simulink model "SAD_testControl"  (R2023b)
settings: Solver=ode8  StartTime=0  StopTime=tf  FixedStep=t_step  RelTol=1e-3
values from neighbouring files (symbols this model uses):
  A_1 = area_face(1)    [SAD_project_code.m]
  A_2 = area_face(2)    [SAD_project_code.m]
  A_3 = area_face(3)    [SAD_project_code.m]
  A_4 = area_face(4)    [SAD_project_code.m]
  A_5 = area_face(5)    [SAD_project_code.m]
  A_6 = area_face(6)    [SAD_project_code.m]
  DCM_eci_per = rotationMatrix(rad2deg(i),rad2deg(OM), rad2deg(om))    [SAD_project_code.m]
  e = 0.0011241    [SAD_project_code.m]
  FS = 50000e-9    (= 5e-05)    [SAD_project_code.m]
  H0 = [g_10 g_11 h_11]'    [SAD_project_code.m]
  h_r_0 = [0,0,0]'    [SAD_project_code.m]
  horizon_cone_limit = deg2rad(70)    [SAD_project_code.m]
  I = 5/12.*diag([Ix Iy Iz])    [SAD_project_code.m]
  i = deg2rad(97.55)    [SAD_project_code.m]
  I_inv = inv(I)    [SAD_project_code.m]
  I_vector_RW = [I_RW I_RW I_RW]'    [SAD_project_code.m]
  inc_tot = sqrt(inc_lin^2 + inc_acc^2)    [SAD_project_code.m]
  InitialTrueAnomalyOfEarth = 0    [SAD_project_code.m]
  j_b = [0.001 0.005 0.001]'    [SAD_project_code.m]
  matrix_RW_config = eye(3)    [SAD_project_code.m]
  matrix_RW_config_inv = inv(matrix_RW_config)    [SAD_project_code.m]
  mu_E = astroConstants(13)    [SAD_project_code.m]
  N_1 = BODY(1,:)    [SAD_project_code.m]
  N_2 = BODY(2,:)    [SAD_project_code.m]
  N_3 = BODY(3,:)    [SAD_project_code.m]
  N_4 = BODY(4,:)    [SAD_project_code.m]
  N_5 = BODY(5,:)    [SAD_project_code.m]
  N_6 = BODY(6,:)    [SAD_project_code.m]
  n_e = sqrt(mu_E/a^3)    [SAD_project_code.m]
  om = deg2rad(206.3209)    [SAD_project_code.m]
  OM = deg2rad(50.7464)    [SAD_project_code.m]
  p = a*(1-e^2)    [SAD_project_code.m]
  q0 = [0.1, -0.7, 0.51, 0.41]    [SAD_project_code.m]
  r_1 = r(1,:)    [SAD_project_code.m]
  r_2 = r(2,:)    [SAD_project_code.m]
  r_3 = r(3,:)    [SAD_project_code.m]
  r_4 = r(4,:)    [SAD_project_code.m]
  r_5 = r(5,:)    [SAD_project_code.m]
  r_6 = r(6,:)    [SAD_project_code.m]
  R_E = astroConstants(23)    [SAD_project_code.m]
  rho_d1 = 0.1    [SAD_project_code.m]
  rho_d2 = 0.1    [SAD_project_code.m]
  rho_d3 = 0.1    [SAD_project_code.m]
  rho_d4 = 0.1    [SAD_project_code.m]
  rho_d5 = 0.1    [SAD_project_code.m]
  rho_d6 = 0.1    [SAD_project_code.m]
  rho_s1 = rho_s(1)    [SAD_project_code.m]
  rho_s2 = rho_s(2)    [SAD_project_code.m]
  rho_s3 = rho_s(3)    [SAD_project_code.m]
  rho_s4 = rho_s(4)    [SAD_project_code.m]
  rho_s5 = rho_s(5)    [SAD_project_code.m]
  rho_s6 = rho_s(6)    [SAD_project_code.m]
  th0 = deg2rad(0)    [SAD_project_code.m]
  ts_sensor = t_step*10    (= 0.1)    [SAD_project_code.m]
  w0 = [wx0 wy0 wz0]'    [SAD_project_code.m]
  w0_RW = [0 0 0]    [SAD_project_code.m]
  w_E = deg2rad(15.04)/60/60    [SAD_project_code.m]
  wMax_RW = 2*pi * RPM_max_RW / 60    (= 527.263967027)    [SAD_project_code.m]
libraries: matrix_library x24, simulink_extras x4, slpidlib x3, sharedtransform x2, simulink x2, vrlib x2, dspinverses x1
(part 1 of 3)
settings Model: Creator=samue  LastModifiedBy=samue

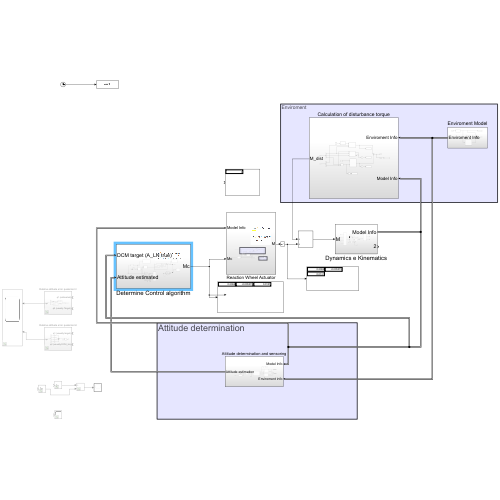
[thumbnail: Simulink's stored preview of the top-level diagram]
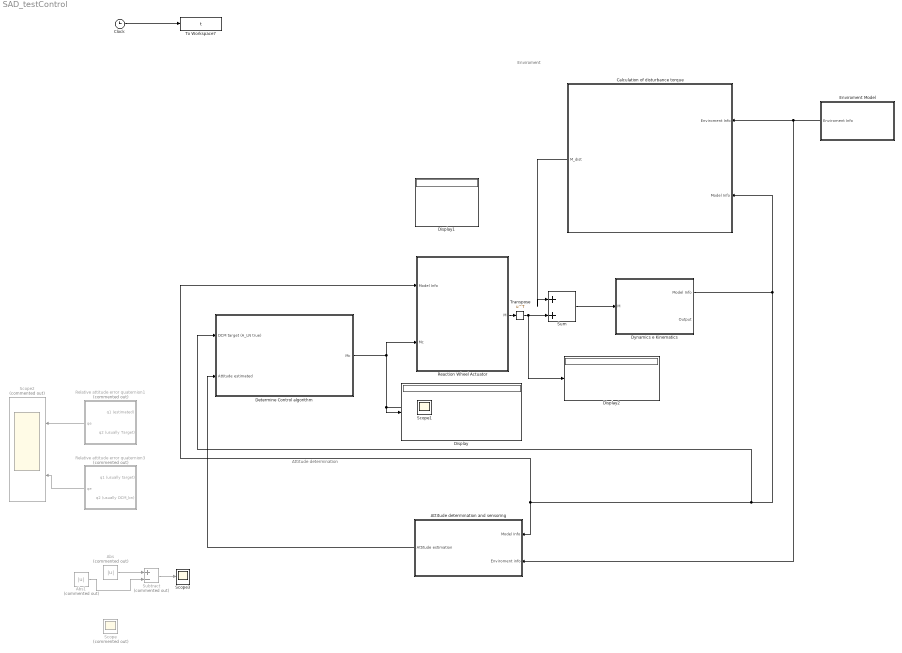
== system SAD_testControl ==
  note: Attitude determination
  note: Enviroment
  Abs : Abs  Commented=on  SaturateOnIntegerOverflow=off
  Abs1 : Abs  Commented=on  SaturateOnIntegerOverflow=off
  Attitude determination and sensoring : Subsystem
  Calculation of disturbance torque : Subsystem
  Clock : Clock
  Determine Control algorithm : Subsystem
  Display : Display
  Display1 : Display
  Display2 : Display
  Dynamics e Kinematics : Subsystem
  Enviroment Model : Subsystem
  Reaction Wheel Actuator : Subsystem
  Relative attitude error quaternion1 : Subsystem  Commented=on
  Relative attitude error quaternion3 : Subsystem  Commented=on
  Scope : Scope  Commented=on
  Scope1 : Scope
  Scope2 : Scope  Commented=on  NumInputPorts=2
  Scope3 : Scope
  Subtract : Sum  Commented=on  Inputs=+-
  Sum : Sum  Inputs=|++
  To Workspace7 : ToWorkspace  VariableName=t  SampleTime=-1
  Transpose : Math  Operator=transpose
  wires:
  Sum/1 -> Dynamics e Kinematics/1(M)
  Enviroment Model/1(Enviroment Info) -> Attitude determination and sensoring/2(Enviroment info), Calculation of disturbance torque/1(Enviroment Info)
  Clock/1 -> To Workspace7/1
  Dynamics e Kinematics/1(Model Info) -> Determine Control algorithm/1(DCM target (A_LN true)), Reaction Wheel Actuator/1(Model Info), Attitude determination and sensoring/1(Model Info), Calculation of disturbance torque/2(Model Info)
  Relative attitude error quaternion3/1(qe) -> Scope2/2
  Abs/1 -> Subtract/1
  Abs1/1 -> Subtract/2
  Subtract/1 -> Scope3/1
  Reaction Wheel Actuator/1(M) -> Transpose/1
  Relative attitude error quaternion1/1(qe) -> Scope2/1
  Attitude determination and sensoring/1(Attitude estimation) -> Determine Control algorithm/2(Attitude estimated)
  Determine Control algorithm/1(Mc) -> Reaction Wheel Actuator/2(Mc), Display/1, Scope1/1
  Transpose/1 -> Display2/1, Sum/2
  Calculation of disturbance torque/1(M_dist) -> Sum/1

== system SAD_testControl/Attitude determination and sensoring ==
  Model Info : Inport
  Enviroment info : Inport  Port=2
  Bus Selector : BusSelector  OutputSignals=B_N,r_n
  Bus Selector1 : BusSelector  OutputSignals=w_b true,DCM_BN
  DCM to quaternion2 : Subsystem
  Horizon Sensor : Subsystem
  MAG-3  Magnetometer1 : Subsystem
  Reshape3 : Reshape
  TRIAD: Attitude determination algebric Method with 2 sensor : Subsystem
  To Workspace5 : ToWorkspace  VariableName=b_sensor  SampleTime=-1
  Transpose : Math  Operator=transpose
  w estimation : Subsystem
  Out Bus Element : Outport  PortName=Attitude estimation  Element=q estimated
  Out Bus Element1 : Outport  PortName=Attitude estimation  Element=DCM_B/N from attirude determination
  Out Bus Element2 : Outport  PortName=Attitude estimation  Element=w estimated
  wires:
  Horizon Sensor/2(R_N Horizon) -> TRIAD: Attitude determination algebric Method with 2 sensor/4(Reference2 (Inertial frame))
  MAG-3  Magnetometer1/1(B_b perturbed sensor) -> TRIAD: Attitude determination algebric Method with 2 sensor/1(Sensor1 (body frame)), Reshape3/1
  DCM to quaternion2/1(q (scalar last)1) -> Out Bus Element/1, w estimation/1(q estimated)  "q estimated"
  w estimation/1(w estimated) -> Out Bus Element2/1  "w estimated"
  Bus Selector/1 -> Transpose/1  "<B_N>"
  Enviroment info/1 -> Bus Selector/1
  Bus Selector/2 -> Horizon Sensor/2(R_N)  "<r_n>"
  Bus Selector1/2 -> Horizon Sensor/1(DCM_B/N), MAG-3  Magnetometer1/1(DCM_B/N)  "<DCM_BN>"
  Reshape3/1 -> To Workspace5/1
  Model Info/1 -> Bus Selector1/1
  Transpose/1 -> MAG-3  Magnetometer1/2(B_N)
  TRIAD: Attitude determination algebric Method with 2 sensor/1(DCM_B/N  Att Det) -> DCM to quaternion2/1(DCM), Out Bus Element1/1
  MAG-3  Magnetometer1/2(B_n) -> TRIAD: Attitude determination algebric Method with 2 sensor/3(Reference1 (Inertial frame))
  Horizon Sensor/1(Perturbed data Horizon) -> TRIAD: Attitude determination algebric Method with 2 sensor/2(Sensor2 (body frame))  "R_b perturbed sensor"

== system SAD_testControl/Calculation of disturbance torque ==
  Enviroment Info : Inport
  Model Info : Inport  Port=2
  Bus Selector : BusSelector  OutputSignals=r_n,S_N,B_N
  Bus Selector1 : BusSelector  OutputSignals=DCM_BL,DCM_BN
  Constant : Constant  Value=I
  Extract Diagonal : matrix_library/Extract Diagonal
      settings: LibrarySourceBlock=|
      | simulink/Matrix
      | Operations/Extract Diagonal
  M of gravity gradient1 : Subsystem
  Magnetic Torque : Subsystem
  Matrix Multiply : Product  Multiplication=Matrix(*)
  Reshape{,1..2,4} (4 alike) : Reshape
  Solar pressure on 6 faces : Subsystem
  Sum : Sum  Inputs=|+++
  Terminator : Terminator
  To Workspace1 : ToWorkspace  VariableName=M_b  SampleTime=-1
  To Workspace2 : ToWorkspace  VariableName=M_dist  SampleTime=-1
  To Workspace3 : ToWorkspace  VariableName=M_GG  SampleTime=-1
  To Workspace6 : ToWorkspace  VariableName=bn  SampleTime=-1
  To Workspace8 : ToWorkspace  VariableName=M_SRP  SampleTime=-1
  j_b : Constant  Value=j_b
  M_dist : Outport
  wires:
  j_b/1 -> Magnetic Torque/1(j_b)
  Magnetic Torque/1(M_b) -> Sum/3, Reshape1/1
  Sum/1 -> Reshape2/1, M_dist/1
  Reshape/1 -> To Workspace8/1
  Reshape1/1 -> To Workspace1/1
  M of gravity gradient1/1(GravityGradient_M) -> To Workspace3/1, Sum/1
  Solar pressure on 6 faces/2(Ftot_SP) -> Terminator/1
  Solar pressure on 6 faces/1(Mtot_SP) -> Reshape/1
  Extract Diagonal/1 -> M of gravity gradient1/1(Inertia Vector)
  Reshape4/1 -> To Workspace6/1
  Matrix Multiply/1 -> Reshape4/1, Magnetic Torque/2(B_b)  "B_b"
  Enviroment Info/1 -> Bus Selector/1
  Constant/1 -> Extract Diagonal/1
  Bus Selector/1 -> M of gravity gradient1/3(r_N), Solar pressure on 6 faces/2("r_N ")  "<r_n>"
  Bus Selector/2 -> Solar pressure on 6 faces/3(S_N)  "<S_N>"
  Bus Selector/3 -> Matrix Multiply/1  "<B_N>"
  Model Info/1 -> Bus Selector1/1
  Bus Selector1/2 -> Matrix Multiply/2, Solar pressure on 6 faces/1(DCM_BN)  "<DCM_BN>"
  Bus Selector1/1 -> M of gravity gradient1/2(A_B/L)  "<DCM_BL>"
  Reshape2/1 -> To Workspace2/1

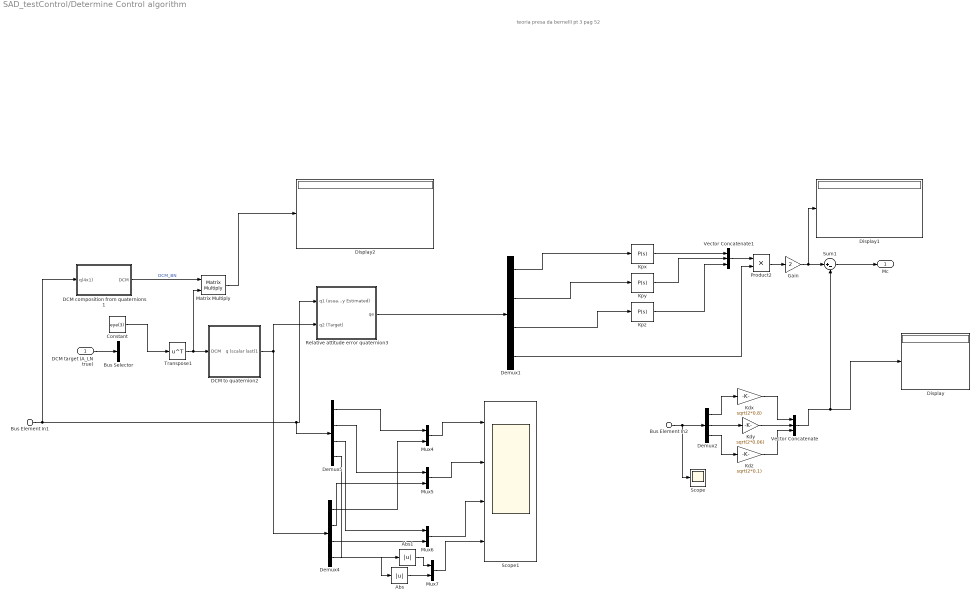
== system SAD_testControl/Determine Control algorithm ==
  note: teoria presa da bernelli pt 3 pag 52
  DCM target (A_LN true) : Inport
  Bus Element In1 : Inport  Port=2  PortName=Attitude estimated  Element=q estimated
  Bus Element In2 : Inport  Port=2  PortName=Attitude estimated  Element=w estimated
  Abs : Abs  SaturateOnIntegerOverflow=off
  Abs1 : Abs  SaturateOnIntegerOverflow=off
  Bus Selector : BusSelector  OutputSignals=A_LN
  Constant : Constant  Value=eye(3)
  DCM composition from quaternions 1 : Subsystem  AncestorBlock=LibrarySAD5/DCM composition from quaternions
  DCM to quaternion2 : Subsystem
  Demux1 : Demux
  Demux2 : Demux  Outputs=3
  Demux4 : Demux
  Demux5 : Demux
  Display : Display
  Display1 : Display
  Display2 : Display
  Gain : Gain  Gain=2
  Kdx : Gain  Gain=sqrt(2*0.8)
  Kdy : Gain  Gain=sqrt(2*0.06)
  Kdz : Gain  Gain=sqrt(2*0.1)
  Kpx : slpidlib/PID Controller  Controller=P  Form=Parallel  TimeDomain=Continuous-time  UseExternalTs=off  SampleTime=5*ts_sensor  IntegratorMethod=Forward Euler  FilterMethod=Forward Euler  ControllerParametersSource=internal  P=0.8  I=-2.93578693683176  UseKiTs=off  D=177.92038615062  N=3.80952380952381  UseFilter=on  TunerSelectOption=Transfer Function Based (PID Tuner App)  InitialConditionSource=internal  InitialConditionForIntegrator=0  InitialConditionForFilter=0  DifferentiatorICPrevScaledInput=0  ExternalReset=none  TrackingMode=off  Kt=1  LimitOutput=off  SatLimitsSource=internal  UpperSaturationLimit=inf  LowerSaturationLimit=-inf  LinearizeAsGain=on  AntiWindupMode=none  Kb=1  LimitIntegrator=off  UpperIntegratorSaturationLimit=inf  LowerIntegratorSaturationLimit=-inf  POutMin=[]  POutMax=[]  IOutMin=[]  IOutMax=[]  DOutMin=[]  DOutMax=[]  NOutMin=[]  NOutMax=[]  SumOutMin=[]  SumOutMax=[]  SaturationOutMin=[]  SaturationOutMax=[]  PParamMin=[]  PParamMax=[]  IParamMin=[]  IParamMax=[]  DParamMin=[]  DParamMax=[]  NParamMin=[]  NParamMax=[]  KbParamMin=[]  KbParamMax=[]  KtParamMin=[]  KtParamMax=[]  KbOutMin=[]  KbOutMax=[]  KtOutMin=[]  KtOutMax=[]  IntegratorOutMin=[]  IntegratorOutMax=[]  FilterOutMin=[]  FilterOutMax=[]  SumI1OutMin=[]  SumI1OutMax=[]  SumI2OutMin=[]  SumI2OutMax=[]  SumI3OutMin=[]  SumI3OutMax=[]  SumI4OutMin=[]  SumI4OutMax=[]  SumDOutMin=[]  SumDOutMax=[]  DifferentiatorOutMin=[]  DifferentiatorOutMax=[]  FilterDiffOutCoefMin=[]  FilterDiffOutCoefMax=[]  ReciprocalOutMin=[]  ReciprocalOutMax=[]  SumDenOutMin=[]  SumDenOutMax=[]  SumNumOutMin=[]  SumNumOutMax=[]  DivideOutMin=[]  DivideOutMax=[]  UdiffTsProdOutMin=[]  UdiffTsProdOutMax=[]  NTsProdOutMin=[]  NTsProdOutMax=[]  UintegralTsProdOutMin=[]  UintegralTsProdOutMax=[]  UngainTsProdOutMin=[]  UngainTsProdOutMax=[]  ClampingZeroOutDataTypeStr=Inherit: Inherit via back propagation  ClampingZeroOutMin=[]  ClampingZeroOutMax=[]  FilterDenConstantOutDataTypeStr=Inherit: Inherit via back propagation  FilterDenConstantOutMin=[]  FilterDenConstantOutMax=[]  PCopyOutDataTypeStr=Inherit: Inherit via back propagation  PCopyOutMin=[]  PCopyOutMax=[]  NCopyOutDataTypeStr=Inherit: Inherit via back propagation  NCopyOutMin=[]  NCopyOutMax=[]  IntegratorContinuousStateAttributes=''  IntegratorStateMustResolveToSignalObject=off  IntegratorRTWStateStorageClass=Auto  FilterContinuousStateAttributes=''  FilterStateMustResolveToSignalObject=off  FilterRTWStateStorageClass=Auto  ParallelPVariant=InternalParameters  IdealPVariant=Disabled  IVariant=Disabled  DVariant=Disabled  IntegratorVariant=Disabled  SatVariant=Disabled  AWVariant=Disabled  PCopyVariant=Disabled  TRVariant=Disabled  FdbkBlocksVariant=Forward  IdealPFdbkVariant=Disabled  SatFdbkVariant=Disabled  DerivativeFilterVariant=Disabled  NVariant=Disabled  NCopyVariant=Disabled_SignalSpec  FilterICVariant=Disabled  IntegratorICVariant=Disabled  ExternalResetVariant=Disabled  TRSumVariant=Passthrough  SumFdbkVariant=Disabled  SumVariant=Passthrough_P  TsampFilterVariant=InternalTs  TsampNgainVariant=Passthrough  TsampIntegralVariant=Disabled_SignalSpec  ExternalSaturationOutDataTypeStr=Inherit: Same as second input
  Kpy : slpidlib/PID Controller  Controller=P  Form=Parallel  TimeDomain=Continuous-time  UseExternalTs=off  SampleTime=5*ts_sensor  IntegratorMethod=Forward Euler  FilterMethod=Forward Euler  ControllerParametersSource=internal  P=0.06  I=-0.105719160910708  UseKiTs=off  D=-16.9301858199188  N=3.80952380952381  UseFilter=on  TunerSelectOption=Transfer Function Based (PID Tuner App)  InitialConditionSource=internal  InitialConditionForIntegrator=0  InitialConditionForFilter=0  DifferentiatorICPrevScaledInput=0  ExternalReset=none  TrackingMode=off  Kt=1  LimitOutput=off  SatLimitsSource=internal  UpperSaturationLimit=inf  LowerSaturationLimit=-inf  LinearizeAsGain=on  AntiWindupMode=none  Kb=1  LimitIntegrator=off  UpperIntegratorSaturationLimit=inf  LowerIntegratorSaturationLimit=-inf  POutMin=[]  POutMax=[]  IOutMin=[]  IOutMax=[]  DOutMin=[]  DOutMax=[]  NOutMin=[]  NOutMax=[]  SumOutMin=[]  SumOutMax=[]  SaturationOutMin=[]  SaturationOutMax=[]  PParamMin=[]  PParamMax=[]  IParamMin=[]  IParamMax=[]  DParamMin=[]  DParamMax=[]  NParamMin=[]  NParamMax=[]  KbParamMin=[]  KbParamMax=[]  KtParamMin=[]  KtParamMax=[]  KbOutMin=[]  KbOutMax=[]  KtOutMin=[]  KtOutMax=[]  IntegratorOutMin=[]  IntegratorOutMax=[]  FilterOutMin=[]  FilterOutMax=[]  SumI1OutMin=[]  SumI1OutMax=[]  SumI2OutMin=[]  SumI2OutMax=[]  SumI3OutMin=[]  SumI3OutMax=[]  SumI4OutMin=[]  SumI4OutMax=[]  SumDOutMin=[]  SumDOutMax=[]  DifferentiatorOutMin=[]  DifferentiatorOutMax=[]  FilterDiffOutCoefMin=[]  FilterDiffOutCoefMax=[]  ReciprocalOutMin=[]  ReciprocalOutMax=[]  SumDenOutMin=[]  SumDenOutMax=[]  SumNumOutMin=[]  SumNumOutMax=[]  DivideOutMin=[]  DivideOutMax=[]  UdiffTsProdOutMin=[]  UdiffTsProdOutMax=[]  NTsProdOutMin=[]  NTsProdOutMax=[]  UintegralTsProdOutMin=[]  UintegralTsProdOutMax=[]  UngainTsProdOutMin=[]  UngainTsProdOutMax=[]  ClampingZeroOutDataTypeStr=Inherit: Inherit via back propagation  ClampingZeroOutMin=[]  ClampingZeroOutMax=[]  FilterDenConstantOutDataTypeStr=Inherit: Inherit via back propagation  FilterDenConstantOutMin=[]  FilterDenConstantOutMax=[]  PCopyOutDataTypeStr=Inherit: Inherit via back propagation  PCopyOutMin=[]  PCopyOutMax=[]  NCopyOutDataTypeStr=Inherit: Inherit via back propagation  NCopyOutMin=[]  NCopyOutMax=[]  IntegratorContinuousStateAttributes=''  IntegratorStateMustResolveToSignalObject=off  IntegratorRTWStateStorageClass=Auto  FilterContinuousStateAttributes=''  FilterStateMustResolveToSignalObject=off  FilterRTWStateStorageClass=Auto  ParallelPVariant=InternalParameters  IdealPVariant=Disabled  IVariant=Disabled  DVariant=Disabled  IntegratorVariant=Disabled  SatVariant=Disabled  AWVariant=Disabled  PCopyVariant=Disabled  TRVariant=Disabled  FdbkBlocksVariant=Forward  IdealPFdbkVariant=Disabled  SatFdbkVariant=Disabled  DerivativeFilterVariant=Disabled  NVariant=Disabled  NCopyVariant=Disabled_SignalSpec  FilterICVariant=Disabled  IntegratorICVariant=Disabled  ExternalResetVariant=Disabled  TRSumVariant=Passthrough  SumFdbkVariant=Disabled  SumVariant=Passthrough_P  TsampFilterVariant=InternalTs  TsampNgainVariant=Passthrough  TsampIntegralVariant=Disabled_SignalSpec  ExternalSaturationOutDataTypeStr=Inherit: Same as second input
  Kpz : slpidlib/PID Controller  Controller=P  Form=Parallel  TimeDomain=Continuous-time  UseExternalTs=off  SampleTime=5*ts_sensor  IntegratorMethod=Forward Euler  FilterMethod=Forward Euler  ControllerParametersSource=internal  P=0.1  I=-0.00390086216682655  UseKiTs=off  D=66.2247876178561  N=3.80952380952381  UseFilter=on  TunerSelectOption=Transfer Function Based (PID Tuner App)  InitialConditionSource=internal  InitialConditionForIntegrator=0  InitialConditionForFilter=0  DifferentiatorICPrevScaledInput=0  ExternalReset=none  TrackingMode=off  Kt=1  LimitOutput=off  SatLimitsSource=internal  UpperSaturationLimit=inf  LowerSaturationLimit=-inf  LinearizeAsGain=on  AntiWindupMode=none  Kb=1  LimitIntegrator=off  UpperIntegratorSaturationLimit=inf  LowerIntegratorSaturationLimit=-inf  POutMin=[]  POutMax=[]  IOutMin=[]  IOutMax=[]  DOutMin=[]  DOutMax=[]  NOutMin=[]  NOutMax=[]  SumOutMin=[]  SumOutMax=[]  SaturationOutMin=[]  SaturationOutMax=[]  PParamMin=[]  PParamMax=[]  IParamMin=[]  IParamMax=[]  DParamMin=[]  DParamMax=[]  NParamMin=[]  NParamMax=[]  KbParamMin=[]  KbParamMax=[]  KtParamMin=[]  KtParamMax=[]  KbOutMin=[]  KbOutMax=[]  KtOutMin=[]  KtOutMax=[]  IntegratorOutMin=[]  IntegratorOutMax=[]  FilterOutMin=[]  FilterOutMax=[]  SumI1OutMin=[]  SumI1OutMax=[]  SumI2OutMin=[]  SumI2OutMax=[]  SumI3OutMin=[]  SumI3OutMax=[]  SumI4OutMin=[]  SumI4OutMax=[]  SumDOutMin=[]  SumDOutMax=[]  DifferentiatorOutMin=[]  DifferentiatorOutMax=[]  FilterDiffOutCoefMin=[]  FilterDiffOutCoefMax=[]  ReciprocalOutMin=[]  ReciprocalOutMax=[]  SumDenOutMin=[]  SumDenOutMax=[]  SumNumOutMin=[]  SumNumOutMax=[]  DivideOutMin=[]  DivideOutMax=[]  UdiffTsProdOutMin=[]  UdiffTsProdOutMax=[]  NTsProdOutMin=[]  NTsProdOutMax=[]  UintegralTsProdOutMin=[]  UintegralTsProdOutMax=[]  UngainTsProdOutMin=[]  UngainTsProdOutMax=[]  ClampingZeroOutDataTypeStr=Inherit: Inherit via back propagation  ClampingZeroOutMin=[]  ClampingZeroOutMax=[]  FilterDenConstantOutDataTypeStr=Inherit: Inherit via back propagation  FilterDenConstantOutMin=[]  FilterDenConstantOutMax=[]  PCopyOutDataTypeStr=Inherit: Inherit via back propagation  PCopyOutMin=[]  PCopyOutMax=[]  NCopyOutDataTypeStr=Inherit: Inherit via back propagation  NCopyOutMin=[]  NCopyOutMax=[]  IntegratorContinuousStateAttributes=''  IntegratorStateMustResolveToSignalObject=off  IntegratorRTWStateStorageClass=Auto  FilterContinuousStateAttributes=''  FilterStateMustResolveToSignalObject=off  FilterRTWStateStorageClass=Auto  ParallelPVariant=InternalParameters  IdealPVariant=Disabled  IVariant=Disabled  DVariant=Disabled  IntegratorVariant=Disabled  SatVariant=Disabled  AWVariant=Disabled  PCopyVariant=Disabled  TRVariant=Disabled  FdbkBlocksVariant=Forward  IdealPFdbkVariant=Disabled  SatFdbkVariant=Disabled  DerivativeFilterVariant=Disabled  NVariant=Disabled  NCopyVariant=Disabled_SignalSpec  FilterICVariant=Disabled  IntegratorICVariant=Disabled  ExternalResetVariant=Disabled  TRSumVariant=Passthrough  SumFdbkVariant=Disabled  SumVariant=Passthrough_P  TsampFilterVariant=InternalTs  TsampNgainVariant=Passthrough  TsampIntegralVariant=Disabled_SignalSpec  ExternalSaturationOutDataTypeStr=Inherit: Same as second input
  Matrix Multiply : Product  Multiplication=Matrix(*)
  Mux{4..7} (4 alike) : Mux  Inputs=2
  Product2 : Product
  Relative attitude error quaternion3 : Subsystem
  Scope : Scope
  Scope1 : Scope  NumInputPorts=4
  Sum1 : Sum  Inputs=|+-
  Transpose1 : Math  Operator=transpose
  Vector Concatenate : Concatenate  NumInputs=3
  Vector Concatenate1 : Concatenate  NumInputs=3
  Mc : Outport
  wires:
  DCM target (A_LN true)/1 -> Bus Selector/1
  Demux4/1 -> Mux4/2
  Demux4/3 -> Mux6/2
  Mux4/1 -> Scope1/1
  Demux4/2 -> Mux5/2
  Demux5/3 -> Mux6/1
  Mux5/1 -> Scope1/2
  Demux5/1 -> Mux4/1
  Bus Element In1/1 -> Demux5/1, Relative attitude error quaternion3/1(q1 (usually Estimated)), DCM composition from quaternions 1/1(q(4x1))
  Mux6/1 -> Scope1/3
  Product2/1 -> Gain/1
  Demux5/2 -> Mux5/1
  Transpose1/1 -> DCM to quaternion2/1(DCM), Matrix Multiply/2
  Mux7/1 -> Scope1/4
  Demux5/4 -> Abs1/1
  Kpx/1 -> Vector Concatenate1/1
  Vector Concatenate1/1 -> Product2/1
  Kpy/1 -> Vector Concatenate1/2
  Kpz/1 -> Vector Concatenate1/3
  Bus Element In2/1 -> Scope/1, Demux2/1
  Demux2/1 -> Kdx/1
  Demux2/2 -> Kdy/1
  Demux2/3 -> Kdz/1
  Kdx/1 -> Vector Concatenate/1
  Kdy/1 -> Vector Concatenate/2
  Kdz/1 -> Vector Concatenate/3
  Vector Concatenate/1 -> Display/1, Sum1/2
  Demux1/1 -> Kpx/1
  Demux1/2 -> Kpy/1
  Demux1/3 -> Kpz/1
  Demux4/4 -> Abs/1
  Gain/1 -> Display1/1, Sum1/1
  Relative attitude error quaternion3/1(qe) -> Demux1/1
  DCM to quaternion2/1(q (scalar last)1) -> Relative attitude error quaternion3/2(q2 (Target)), Demux4/1
  Abs/1 -> Mux7/2
  Abs1/1 -> Mux7/1
  Sum1/1 -> Mc/1
  Demux1/4 -> Product2/2
  DCM composition from quaternions 1/1(DCM) -> Matrix Multiply/1  "DCM_BN"
  Matrix Multiply/1 -> Display2/1
  Constant/1 -> Transpose1/1

== system SAD_testControl/Dynamics e Kinematics ==
  M : Inport
  Attitude error GG : Subsystem
  Constant : Constant  Value=I_inv
  Constant6 : Constant  Value=q0
  DCM composition from quaternions 1 : Subsystem  AncestorBlock=LibrarySAD5/DCM composition from quaternions
  Inertia Matrix : Constant  Value=I  VectorParams1D=off
  Initial Condition W : Constant  Value=w0
  Kinematics quaternion2 : Subsystem
  Reshape : Reshape
  Reshape1 : Reshape
  Scope : Scope
  Single spin dynamics : Subsystem  AncestorBlock=My_library/Single spin dynamics
  Terminator1 : Terminator
  To Workspace2 : ToWorkspace  VariableName=wb  SampleTime=-1
  To Workspace4 : ToWorkspace  VariableName=w  SampleTime=-1
  Out Bus Element : Outport  PortName=Model Info  Element=w_b true
  Out Bus Element1 : Outport  PortName=Model Info  Element=Ang vel error
  Out Bus Element2 : Outport  PortName=Model Info  Element=DCM_BL
  Out Bus Element3 : Outport  PortName=Model Info  Element=q_b True
  Out Bus Element4 : Outport  PortName=Model Info  Element=DCM_BN
  Out Bus Element5 : Outport  PortName=Model Info  Element=A_LN
  Output : Outport  Port=2
  wires:
  Single spin dynamics/1(Omega) -> Scope/1, Out Bus Element/1, Attitude error GG/1(w), Reshape1/1, Kinematics quaternion2/1(omega)  "w_b true"
  M/1 -> Single spin dynamics/4(M)
  Constant/1 -> Single spin dynamics/1(Inertia matrix inverse)
  Inertia Matrix/1 -> Single spin dynamics/2(Inertia matrix)
  Initial Condition W/1 -> Single spin dynamics/3(Omega_0)
  Constant6/1 -> Kinematics quaternion2/2(q0)
  Kinematics quaternion2/1(q) -> DCM composition from quaternions 1/1(q(4x1)), Output/1, Out Bus Element3/1  "q_b True"
  Reshape1/1 -> To Workspace4/1
  Kinematics quaternion2/2(q^(-1)) -> Terminator1/1
  DCM composition from quaternions 1/1(DCM) -> Out Bus Element4/1, Attitude error GG/2(DCM_B/N)  "DCM_BN"
  Attitude error GG/1(Ang Vel Error) -> Out Bus Element1/1, Reshape/1  "Ang vel error"
  Attitude error GG/2(DCM_B/L) -> Out Bus Element2/1
  Reshape/1 -> To Workspace2/1
  Attitude error GG/3(A_L/N) -> Out Bus Element5/1

== system SAD_testControl/Enviroment Model ==
  Bus Creator : BusCreator  Inputs=3
  Constant4 : Constant  Value=th0
  Magnetic Field : Subsystem
  Sun Position in Earth Centred Equatorial Inertial RF : Subsystem
  To Workspace : ToWorkspace  VariableName=r_n  SampleTime=-1
  two-body Keplerian dynamics ECI : Subsystem
  Enviroment Info : Outport
  wires:
  Constant4/1 -> two-body Keplerian dynamics ECI/1(th0)
  Sun Position in Earth Centred Equatorial Inertial RF/1(s_N) -> Bus Creator/2  "S_N"
  two-body Keplerian dynamics ECI/1(r_n) -> Magnetic Field/1(r_N), Bus Creator/1, To Workspace/1  "r_n"
  Magnetic Field/1(B_N) -> Bus Creator/3  "B_N"
  Bus Creator/1 -> Enviroment Info/1

== system SAD_testControl/Reaction Wheel Actuator ==
  note: W integration
  note: MAIN INTEGRATION
  BusElementIn : Inport  PortName=Model Info  Element=w_b true
  Mc : Inport  Port=2
  Calculatate wRW in base of saturation : Subsystem
  Constant3 : Constant  Value=I_vector_RW
  Constant5 : Constant  Value=h_r_0  VectorParams1D=off
  Constant6 : Constant  Value=matrix_RW_config  VectorParams1D=off
  Constant8 : Constant  Value=matrix_RW_config_inv  VectorParams1D=off
  Constant9 : Constant  Value=w0_RW
  Cross Product : matrix_library/Cross Product
  Divide : Product  Inputs=*/
  Gain : Gain  Gain=-1
  Integrator : Integrator  InitialConditionSource=external
  Integrator1 : Integrator  InitialConditionSource=external
  Matrix Multiply : Product  Multiplication=Matrix(*)
  Matrix Multiply1 : Product  Multiplication=Matrix(*)
  Reshape : Reshape
  Reshape4 : Reshape
  Subsystem1 : Subsystem
  Sum : Sum  Inputs=|++
  To Workspace1 : ToWorkspace  VariableName=wr  SampleTime=-1
  To Workspace6 : ToWorkspace  VariableName=T_rotor  SampleTime=-1
  Transpose : Math  Operator=transpose
  detect if the RW is saturated (output == 1 isSaturated) : Subsystem
  M : Outport
  wires:
  Matrix Multiply1/1 -> Reshape4/1, Integrator/1, Divide/1  "h_r dot"
  Constant6/1 -> Matrix Multiply/1
  Cross Product/1 -> Sum/2
  Constant8/1 -> Gain/1
  Sum/1 -> Matrix Multiply1/2
  detect if the RW is saturated (output == 1 isSaturated)/2(flag RW2) -> Calculatate wRW in base of saturation/3(flag RW2 (1 is saturated)), Subsystem1/2(flag RW2 (1 is saturated))  "flag RW2 (1 is saturated)"
  Calculatate wRW in base of saturation/1(wRW) -> Reshape/1
  Matrix Multiply/1 -> Cross Product/2
  Constant5/1 -> Integrator/2
  Constant3/1 -> Divide/2
  Gain/1 -> Matrix Multiply1/1
  Mc/1 -> Subsystem1/4(Mc), Sum/1
  Integrator1/1 -> Calculatate wRW in base of saturation/1(wRW integrated), detect if the RW is saturated (output == 1 isSaturated)/1(w)  "wRW integrated"
  Constant9/1 -> Integrator1/2
  Divide/1 -> Integrator1/1  "wRW dot"
  Integrator/1 -> Matrix Multiply/2  "h_r"
  detect if the RW is saturated (output == 1 isSaturated)/3(flag RW3) -> Calculatate wRW in base of saturation/4(flag RW3 (1 is saturated)), Subsystem1/3(flag RW3 (1 is saturated))  "flag RW3 (1 is saturated)"
  detect if the RW is saturated (output == 1 isSaturated)/1(flag RW1) -> Calculatate wRW in base of saturation/2(flag RW1 (1 is saturated)), Subsystem1/1(flag RW1 (1 is saturated))  "flag RW1 (1 is saturated)"
  Reshape/1 -> To Workspace1/1
  BusElementIn/1 -> Transpose/1
  Transpose/1 -> Cross Product/1
  Subsystem1/1(M) -> M/1
  Reshape4/1 -> To Workspace6/1

== system SAD_testControl/Relative attitude error quaternion1 ==
  q1 (estimated) : Inport
  q2 (usually Target) : Inport  Port=2
  Create Diagonal Matrix : matrix_library/Create Diagonal Matrix
      settings: LibrarySourceBlock=|
      | simulink/Matrix
      | Operations/Create Diagonal
      | Matrix
  Create Diagonal Matrix1 : matrix_library/Create Diagonal Matrix
      settings: LibrarySourceBlock=|
      | simulink/Matrix
      | Operations/Create Diagonal
      | Matrix
  Demux : Demux
  Gain2 : Gain  Gain=-1
  Matrix Concatenate : Concatenate  Mode=Multidimensional array  ConcatenateDimension=2
  Matrix Concatenate1 : Concatenate  Mode=Multidimensional array
  Matrix Multiply : Product  Multiplication=Matrix(*)
  Subtract : Sum  Inputs=+-
  Transpose : Math  Operator=transpose
  Vector Concatenate : Concatenate  NumInputs=3
  Vector Concatenate1 : Concatenate
  qe : Outport
  wires:
  Demux/2 -> Vector Concatenate/2
  Demux/1 -> Vector Concatenate/1
  Demux/3 -> Vector Concatenate/3
  Demux/4 -> Create Diagonal Matrix1/1, Vector Concatenate1/2
  q2 (usually Target)/1 -> Matrix Multiply/2
  Matrix Multiply/1 -> qe/1
  q1 (estimated)/1 -> Demux/1
  Subtract/1 -> Matrix Concatenate/1
  Gain2/1 -> Matrix Concatenate/2
  Matrix Concatenate/1 -> Matrix Concatenate1/1
  Vector Concatenate1/1 -> Transpose/1
  Transpose/1 -> Matrix Concatenate1/2
  Matrix Concatenate1/1 -> Matrix Multiply/1
  Create Diagonal Matrix1/1 -> Subtract/1
  Vector Concatenate/1 -> Create Diagonal Matrix/1, Vector Concatenate1/1, Gain2/1
  Create Diagonal Matrix/1 -> Subtract/2

== system SAD_testControl/Relative attitude error quaternion3 ==
  q1 (usually target) : Inport
  q2 (usually DCM_bn) : Inport  Port=2
  Demux : Demux
  Gain1 : Gain  Gain=[0,0,0,-1; 0,0,1,0; 0,-1,0 0; 1,0,0,0]
  Gain2 : Gain  Gain=[0, 0, -1 ,0; 0, 0 ,0 ,-1; 1, 0, 0, 0; 0 1, 0, 0]
  Gain3 : Gain  Gain=[0 1 0 0; -1 0 0 0; 0 0 0 -1; 0 0 1 0]
  Gain4 : Gain  Gain=eye(4)
  Matrix Multiply : Product  Multiplication=Matrix(*)
  Sum1 : Sum  Inputs=++++
  qe : Outport
  wires:
  Gain1/1 -> Sum1/1
  Demux/2 -> Gain2/1
  Gain3/1 -> Sum1/3
  Demux/1 -> Gain1/1
  Sum1/1 -> Matrix Multiply/1
  Demux/3 -> Gain3/1
  Gain4/1 -> Sum1/4
  Gain2/1 -> Sum1/2
  Demux/4 -> Gain4/1
  q2 (usually DCM_bn)/1 -> Matrix Multiply/2
  Matrix Multiply/1 -> qe/1
  q1 (usually target)/1 -> Demux/1

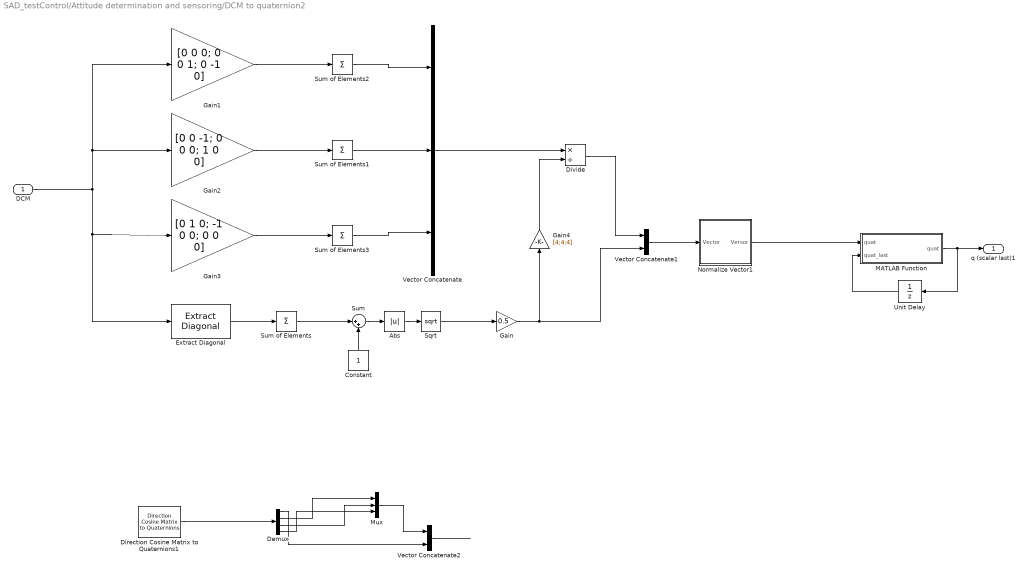
== system SAD_testControl/Attitude determination and sensoring/DCM to quaternion2 ==
  DCM : Inport
  Abs : Abs  SaturateOnIntegerOverflow=off
  Constant : Constant
  Demux : Demux
  Direction Cosine Matrix to Quaternions1 : sharedtransform/Direction Cosine Matrix  to Quaternions  aMode=0  action=None  tolerance=eps(2)
      settings: LibrarySourceBlock=|
      | aerolibtransform2/Direction Cosine Matrix
      | to Quaternions
  Divide : Product  Inputs=*/
  Extract Diagonal : matrix_library/Extract Diagonal
      settings: LibrarySourceBlock=|
      | simulink/Matrix
      | Operations/Extract Diagonal
  Gain : Gain  Gain=0.5
  Gain1 : Gain  Gain=[0 0 0; 0 0 1; 0 -1 0]
  Gain2 : Gain  Gain=[0 0 -1; 0 0 0; 1 0 0]
  Gain3 : Gain  Gain=[0 1 0; -1 0 0; 0 0 0]
  Gain4 : Gain  Gain=[4;4;4]
  MATLAB Function : MATLAB Function  TreatAsAtomicUnit=on
  Mux : Mux  Inputs=3
  Normalize Vector1 : Subsystem
  Sqrt : Sqrt
  Sum : Sum  Inputs=|++
  Sum of Elements{,1..3} (4 alike) : Sum  Inputs=+
  Unit Delay : UnitDelay  InitialCondition=q0  SampleTime=-1  HasFrameUpgradeWarning=on
  Vector Concatenate : Concatenate  NumInputs=3
  Vector Concatenate1 : Concatenate
  Vector Concatenate2 : Concatenate
  q (scalar last)1 : Outport
  wires:
  Extract Diagonal/1 -> Sum of Elements/1
  Sum of Elements/1 -> Sum/1
  Constant/1 -> Sum/2
  Sqrt/1 -> Gain/1
  DCM/1 -> Gain1/1, Gain2/1, Gain3/1, Extract Diagonal/1
  Gain2/1 -> Sum of Elements1/1
  Sum of Elements1/1 -> Vector Concatenate/2
  Gain1/1 -> Sum of Elements2/1
  Sum of Elements2/1 -> Vector Concatenate/1
  Sum of Elements3/1 -> Vector Concatenate/3
  Gain3/1 -> Sum of Elements3/1
  Vector Concatenate/1 -> Divide/1
  Gain/1 -> Vector Concatenate1/2, Gain4/1
  Divide/1 -> Vector Concatenate1/1
  Vector Concatenate1/1 -> Normalize Vector1/1(Vector)
  Normalize Vector1/1(Versor) -> MATLAB Function/1("quat ")
  Sum/1 -> Abs/1
  Gain4/1 -> Divide/2
  Abs/1 -> Sqrt/1
  Direction Cosine Matrix to Quaternions1/1 -> Demux/1
  Demux/2 -> Mux/1
  Demux/3 -> Mux/2
  Demux/4 -> Mux/3
  Demux/1 -> Vector Concatenate2/2
  Mux/1 -> Vector Concatenate2/1
  Vector Concatenate2/1 -> ?
  ? -> Direction Cosine Matrix to Quaternions1/1
  Unit Delay/1 -> MATLAB Function/2(quat_last)
  MATLAB Function/1(quat) -> Unit Delay/1, q (scalar last)1/1

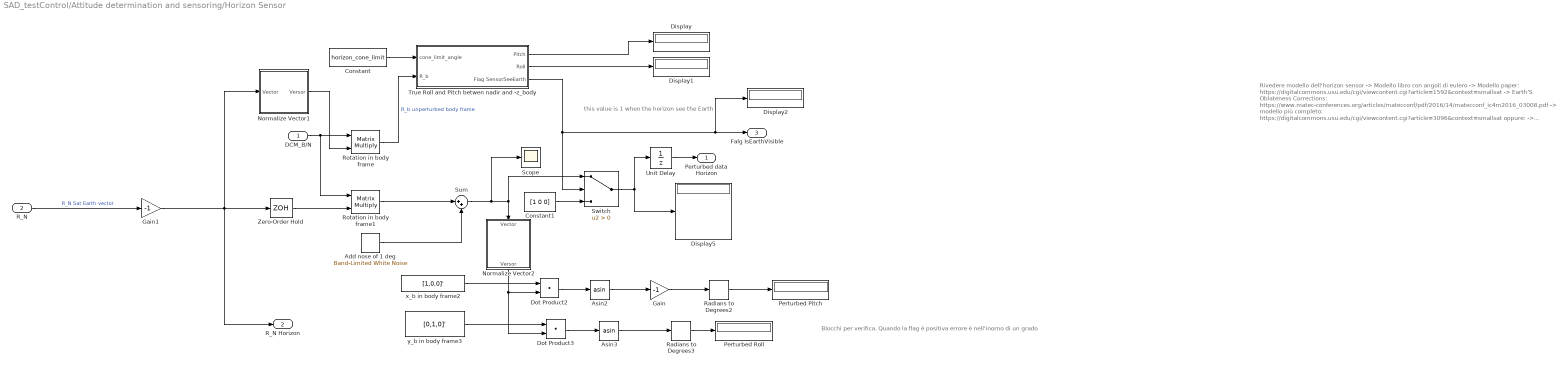
== system SAD_testControl/Attitude determination and sensoring/Horizon Sensor ==
  note: this value is 1 when the horizon see the Earth
  note: Rivedere modello dell'horizon sensor
      | -> Modello libro con angoli di eulero
      | -> Modello paper: https://digitalcommons.usu.edu/cgi/viewcontent.cgi?article=1592&context=smallsat
      | -> Earth’S Oblateness Corrections: https://www.matec-conferences.org/articles/matecconf/pdf/2016/14/matecconf_ic4m2016_03008.pdf
      | -> modello più completo: https://digitalcommons.usu.edu/cgi/viewcontent.cgi?article=3096&context=smallsat
      | oppure:
      | -> Sistemare errore in modo che non sia lineare
      | -> Controllare angoli e conversioni
  note: Blocchi per verifica. Quando la flag è positiva errore è nell'inorno di un grado
  DCM_B/N : Inport
  R_N : Inport  Port=2
  Add nose of 1 deg : simulink/Sources/Band-Limited White Noise  Cov=[0.00001 0.00001 0]  Ts=ts_sensor  seed=[23341]
  Asin2 : Trigonometry  Operator=asin
  Asin3 : Trigonometry  Operator=asin
  Constant : Constant  Value=horizon_cone_limit
  Constant1 : Constant  Value=[1 0 0]
  Display{,1..2,5} (4 alike) : Display
  Dot Product2 : DotProduct  OutDataTypeStr=Inherit: Inherit via internal rule
  Dot Product3 : DotProduct  OutDataTypeStr=Inherit: Inherit via internal rule
  Gain : Gain  Gain=-1
  Gain1 : Gain  Gain=-1
  Normalize Vector1 : Subsystem
  Normalize Vector2 : Subsystem
  Perturbed Pitch : Display
  Perturbed Roll : Display
  Radians to Degrees2 : simulink_extras/Transformations/Radians to Degrees
  Radians to Degrees3 : simulink_extras/Transformations/Radians to Degrees
  Rotation in body frame : Product  Multiplication=Matrix(*)
  Rotation in body frame1 : Product  Multiplication=Matrix(*)
  Scope : Scope
  Sum : Sum  Inputs=|++
  Switch : Switch  Criteria=u2 > Threshold  SaturateOnIntegerOverflow=off  InputSameDT=off
  True Roll and Pitch betwen nadir and -z_body : Subsystem
  Unit Delay : UnitDelay  InitialCondition=[0 1 0]'  SampleTime=-1  HasFrameUpgradeWarning=on
  Zero-Order Hold : ZeroOrderHold  SampleTime=ts_sensor
  x_b in body frame2 : Constant  Value=[1,0,0]'
  y_b in body frame3 : Constant  Value=[0,1,0]'
  Perturbed data Horizon : Outport
  R_N Horizon : Outport  Port=2
  Falg IsEarthVisible : Outport  Port=3
  wires:
  y_b in body frame3/1 -> Dot Product3/1
  Zero-Order Hold/1 -> Rotation in body frame1/2
  True Roll and Pitch betwen nadir and -z_body/3(Flag SensorSeeEarth) -> Falg IsEarthVisible/1, Display2/1, Switch/2
  Normalize Vector1/1(Versor) -> Rotation in body frame/2
  Rotation in body frame1/1 -> Sum/1
  Asin2/1 -> Gain/1
  DCM_B/N/1 -> Rotation in body frame/1, Rotation in body frame1/1
  Switch/1 -> Unit Delay/1, Display5/1
  True Roll and Pitch betwen nadir and -z_body/1(Pitch) -> Display/1
  Constant/1 -> True Roll and Pitch betwen nadir and -z_body/1(cone_limit_angle)
  Dot Product2/1 -> Asin2/1
  Rotation in body frame/1 -> True Roll and Pitch betwen nadir and -z_body/2(R_b)  "R_b unperturbed body frame"
  Add nose of 1 deg/1 -> Sum/2
  True Roll and Pitch betwen nadir and -z_body/2(Roll) -> Display1/1
  x_b in body frame2/1 -> Dot Product2/1
  Radians to Degrees2/1 -> Perturbed Pitch/1
  Sum/1 -> Scope/1, Switch/1, Normalize Vector2/1(Vector)
  Dot Product3/1 -> Asin3/1
  Asin3/1 -> Radians to Degrees3/1
  Gain/1 -> Radians to Degrees2/1
  Radians to Degrees3/1 -> Perturbed Roll/1
  Constant1/1 -> Switch/3
  R_N/1 -> Gain1/1  "R_N Sat Earth vector"
  Normalize Vector2/1(Versor) -> Dot Product2/2, Dot Product3/2
  Gain1/1 -> Zero-Order Hold/1, Normalize Vector1/1(Vector), R_N Horizon/1
  Unit Delay/1 -> Perturbed data Horizon/1

== system SAD_testControl/Attitude determination and sensoring/MAG-3  Magnetometer1 ==
  note: CODE TO ADD TO MAKE SENSOR WORK
      | % Time definition
      | t0 = 0;
      | tf = T; %Period of orbit
      | t_step = 0.01; %fixed step of simulation
      | ts_sensor = t_step; % Sample of sensor (can change but must to be a multiple of t_step)
      |
      | % MAG-3 sensor data and error
      | FS = 500e-9; %Full scale value
      | inc_lin = 0.15/100; % Accuracy error
      | inc_acc = 0.75/100; % Linear error
      | inc_tot = sqrt(inc_lin^2 + inc_acc^2); %Total error
  DCM_B/N : Inport
  B_N : Inport  Port=2
  Error gain of sensor MAG-3 : Gain  Gain=inc_tot*FS
  Rotation in body frame : Product  Multiplication=Matrix(*)
  Saturation to FS : Saturate  UpperLimit=FS  LowerLimit=-FS
  Sum : Sum  Inputs=|++
  Unit Delay : UnitDelay  InitialCondition=[0,0,1]'  SampleTime=-1  HasFrameUpgradeWarning=on
  Vector Concatenate : Concatenate  NumInputs=3
  White Noise : RandomNumber  DisableCoverage=on  Seed=1  SampleTime=ts_sensor
  White Noise1 : RandomNumber  DisableCoverage=on  Seed=2  SampleTime=ts_sensor
  White Noise2 : RandomNumber  DisableCoverage=on  Seed=3  SampleTime=ts_sensor
  Zero-Order Hold : ZeroOrderHold  SampleTime=ts_sensor
  B_b perturbed sensor : Outport
  B_n : Outport  Port=2
  wires:
  Vector Concatenate/1 -> Error gain of sensor MAG-3/1
  White Noise/1 -> Vector Concatenate/1
  Error gain of sensor MAG-3/1 -> Sum/2
  White Noise2/1 -> Vector Concatenate/3
  White Noise1/1 -> Vector Concatenate/2
  DCM_B/N/1 -> Rotation in body frame/1
  B_N/1 -> B_n/1, Zero-Order Hold/1
  Saturation to FS/1 -> Unit Delay/1
  Rotation in body frame/1 -> Sum/1
  Sum/1 -> Saturation to FS/1
  Zero-Order Hold/1 -> Rotation in body frame/2
  Unit Delay/1 -> B_b perturbed sensor/1

== system SAD_testControl/Attitude determination and sensoring/TRIAD: Attitude determination algebric Method with 2 sensor ==
  note: 𝑉^(-1) = 𝑉';
      | 𝐴 = 𝑆𝑉^(-1) = 𝑆𝑉'
  note: 𝑣1 = 𝑎;
      | 𝑣2 = (𝑎 ∧ 𝑏)/|𝑎 ∧ 𝑏|;
      | 𝑣3 = 𝑎 ∧ 𝑣2
  note: S1 = 𝑝;
      | 𝑠2 = (𝑝 ∧ 𝑞)/(|𝑝 ∧ 𝑞|);
      | 𝑠3 = 𝑝 ∧ 𝑠2
  Sensor1 (body frame) : Inport
  Sensor2 (body frame) : Inport  Port=2
  Reference1 (Inertial frame) : Inport  Port=3
  Reference2 (Inertial frame) : Inport  Port=4
  Matrix Multiply : Product  Multiplication=Matrix(*)
  Normalize Vector1 : Subsystem
  Normalize Vector2 : Subsystem
  Normalize Vector3 : Subsystem
  Normalize Vector4 : Subsystem
  Subsystem : Subsystem
  Subsystem1 : Subsystem
  Transpose : Math  Operator=transpose
  DCM_B/N  Att Det : Outport
  wires:
  Sensor1 (body frame)/1 -> Normalize Vector2/1(Vector)  "q"
  Sensor2 (body frame)/1 -> Normalize Vector3/1(Vector)  "p"
  Subsystem/1("Matrix S Measurements ") -> Matrix Multiply/1  "Matrix S Measurements (body frame)"
  Normalize Vector2/1(Versor) -> Subsystem/1(versor p (body frame))
  Normalize Vector3/1(Versor) -> Subsystem/2(versor q (body frame))
  Reference2 (Inertial frame)/1 -> Normalize Vector4/1(Vector)  "b"
  Reference1 (Inertial frame)/1 -> Normalize Vector1/1(Vector)  "a"
  Subsystem1/1("Matrix V certain model ") -> Transpose/1  "Matrix V (inertial frame)"
  Normalize Vector4/1(Versor) -> Subsystem1/2(versor b (inertial))
  Matrix Multiply/1 -> DCM_B/N  Att Det/1  "DCM_B/N from attirude determination"
  Transpose/1 -> Matrix Multiply/2
  Normalize Vector1/1(Versor) -> Subsystem1/1(versor a (inertial))

== system SAD_testControl/Attitude determination and sensoring/w estimation ==
  q estimated : Inport
  Demux : Demux
  Derivative : Derivative
  Gain : Gain  Gain=[0,0,0; 0,0,-1; 0 1, 0;-1,0,0]
  Gain1 : Gain  Gain=[0,0,1;0,0,0;-1,0,0;0,-1,0]
  Gain2 : Gain  Gain=[0,-1,0;1,0,0;0,0,0;0,0,-1]
  Gain3 : Gain  Gain=[1,0,0;0,1,0;0,0,1;0,0,0]
  Gain4 : Gain  Gain=2
  Matrix Multiply : Product  Multiplication=Matrix(*)
  Pseudoinverse : dspinverses/Pseudoinverse  wanterr=off  SimulateUsing=Interpreted execution
  Sum : Sum  Inputs=|++++
  w estimated : Outport
  wires:
  Matrix Multiply/1 -> Gain4/1
  Derivative/1 -> Matrix Multiply/2
  Pseudoinverse/1 -> Matrix Multiply/1
  Demux/3 -> Gain2/1
  Gain1/1 -> Sum/2
  q estimated/1 -> Demux/1, Derivative/1
  Sum/1 -> Pseudoinverse/1
  Demux/2 -> Gain1/1
  Gain3/1 -> Sum/4
  Demux/4 -> Gain3/1
  Gain2/1 -> Sum/3
  Demux/1 -> Gain/1
  Gain/1 -> Sum/1
  Gain4/1 -> w estimated/1

== system SAD_testControl/Calculation of disturbance torque/M of gravity gradient1 ==
  Inertia Vector : Inport
  A_B/L : Inport  Port=2
  r_N : Inport  Port=3
  Constant : Constant  Value=3
  Constant11 : Constant  Value=[1,0,0]
  Demux1 : Demux  Outputs=3
  Divide : Product  Inputs=*/
  Gain : Gain  Gain=3*mu_E
  Gain1 : Gain  Gain=[0;-1;1]
  Gain2 : Gain  Gain=[1;0;-1]
  Gain3 : Gain  Gain=[-1;1;0]
  Matrix Multiply2 : Product  Multiplication=Matrix(*)
  Norm of vector : Subsystem  AncestorBlock=LibrarySAD5/Normalize Vector1
  Power : Math  Operator=pow
  Product2 : Product  Inputs=3
  Product3 : Product  Inputs=3
  Product4 : Product  Inputs=3
  Scope : Scope
  Sum of Elements : Sum  Inputs=+
  Sum of Elements1 : Sum  Inputs=+
  Sum of Elements2 : Sum  Inputs=+
  Vector Concatenate4 : Concatenate  NumInputs=3
  GravityGradient_M : Outport
  wires:
  Demux1/3 -> Product2/3, Product3/3
  Product2/1 -> Vector Concatenate4/1
  Matrix Multiply2/1 -> Demux1/1
  Product4/1 -> Vector Concatenate4/3
  Product3/1 -> Vector Concatenate4/2
  Demux1/1 -> Product4/2, Product3/2
  Constant11/1 -> Matrix Multiply2/2
  Demux1/2 -> Product4/3, Product2/2
  A_B/L/1 -> Matrix Multiply2/1
  Vector Concatenate4/1 -> Gain/1
  Gain1/1 -> Sum of Elements/1
  Gain2/1 -> Sum of Elements1/1
  Gain3/1 -> Sum of Elements2/1
  Sum of Elements/1 -> Product2/1
  Sum of Elements1/1 -> Product3/1
  Sum of Elements2/1 -> Product4/1
  Inertia Vector/1 -> Gain1/1, Gain2/1, Gain3/1
  Gain/1 -> Divide/1
  Power/1 -> Scope/1, Divide/2
  Constant/1 -> Power/2
  r_N/1 -> Norm of vector/1(Vector)
  Divide/1 -> GravityGradient_M/1
  Norm of vector/1(Norm) -> Power/1

== system SAD_testControl/Calculation of disturbance torque/Magnetic Torque ==
  j_b : Inport
  B_b : Inport  Port=2
  Cross Product : matrix_library/Cross Product
  M_b : Outport
  wires:
  Cross Product/1 -> M_b/1
  j_b/1 -> Cross Product/1
  B_b/1 -> Cross Product/2

== system SAD_testControl/Calculation of disturbance torque/Solar pressure on 6 faces ==
  DCM_BN : Inport
  "r_N " : Inport  Port=2
  S_N : Inport  Port=3
  Acos : Trigonometry  Operator=acos
  Dot Product : DotProduct  OutDataTypeStr=Inherit: Inherit via internal rule
  MatrixMultiply : Product  Multiplication=Matrix(*)
  MatrixMultiply1 : Product  Multiplication=Matrix(*)
  Norm of vector : Subsystem  AncestorBlock=LibrarySAD5/Normalize Vector1
  Normalize Vector : vrlib/Utilities/Normalize Vector  maxzero=0
  Normalize Vector1 : vrlib/Utilities/Normalize Vector  maxzero=0
  Solar pressure on 6 faces1 : Subsystem
  Sum1 : Sum  Inputs=|+-
  Mtot_SP : Outport
  Ftot_SP : Outport  Port=2
  wires:
  DCM_BN/1 -> MatrixMultiply1/1, MatrixMultiply/1
  S_N/1 -> Norm of vector/1(Vector), Sum1/1, MatrixMultiply/2, Normalize Vector1/1
  "r_N "/1 -> Sum1/2, MatrixMultiply1/2
  MatrixMultiply1/1 -> Solar pressure on 6 faces1/2(r_B)
  Norm of vector/1(Norm) -> Solar pressure on 6 faces1/5(s_N norm)
  MatrixMultiply/1 -> Solar pressure on 6 faces1/1(s_B)
  Sum1/1 -> Solar pressure on 6 faces1/4(S_N - r_N), Normalize Vector/1
  Normalize Vector/1 -> Dot Product/1
  Normalize Vector1/1 -> Dot Product/2
  Solar pressure on 6 faces1/1(Ftot_SP) -> Ftot_SP/1
  Dot Product/1 -> Acos/1
  Acos/1 -> Solar pressure on 6 faces1/3(S/E_S/sc_angle)
  Solar pressure on 6 faces1/2(Mtot_SP) -> Mtot_SP/1

== system SAD_testControl/Determine Control algorithm/DCM composition from quaternions 1 ==
  q(4x1) : Inport
  Cross product matrix composition : Subsystem
  Demux : Demux
  Dot Product : DotProduct  OutDataTypeStr=Inherit: Inherit via internal rule
  Gain : Gain  Gain=[1 0 0; 0 1 0; 0 0 1]
  Gain1 : Gain  Gain=2
  Gain2 : Gain  Gain=-2
  Mux : Mux  Inputs=3
  Product : Product  Multiplication=Matrix(*)
  Product1 : Product
  Square : Math  Operator=square
  Sum : Sum  Inputs=|-+
  Sum1 : Sum  Inputs=+++
  Transpose : Math  Operator=transpose
  DCM : Outport
  wires:
  Gain/1 -> Sum1/1
  Demux/1 -> Mux/1
  q(4x1)/1 -> Demux/1
  Demux/2 -> Mux/2
  Mux/1 -> Dot Product/2, Dot Product/1, Product/1, Cross product matrix composition/1(q_vect), Transpose/1  "q_vect"
  Demux/4 -> Gain2/1, Square/1  "q4"
  Demux/3 -> Mux/3
  Dot Product/1 -> Sum/1
  Sum/1 -> Gain/1
  Square/1 -> Sum/2
  Transpose/1 -> Product/2
  Product/1 -> Gain1/1
  Gain2/1 -> Product1/2
  Cross product matrix composition/1(q_vect cross) -> Product1/1  "omega_mat"
  Product1/1 -> Sum1/3
  Gain1/1 -> Sum1/2
  Sum1/1 -> DCM/1

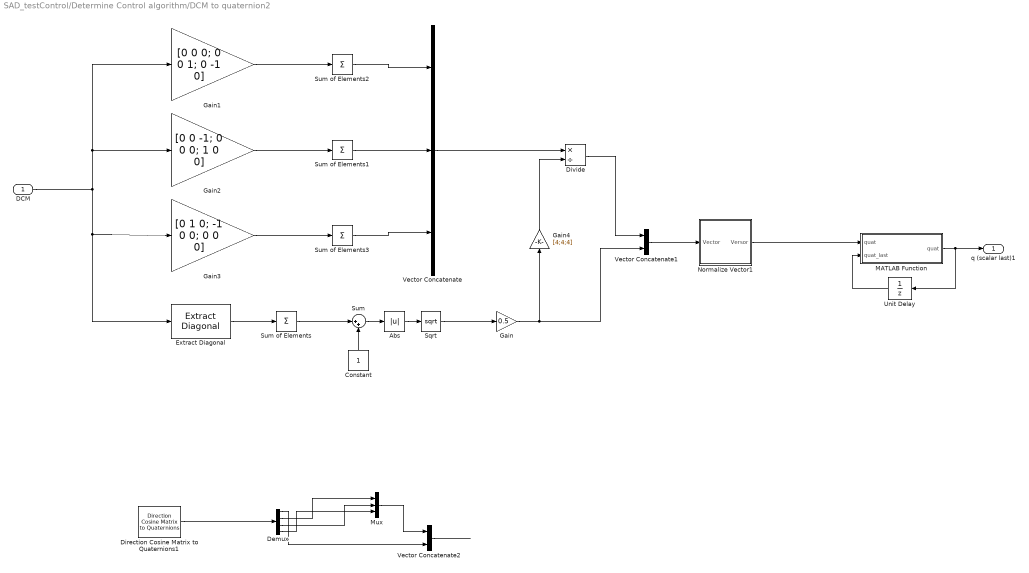
== system SAD_testControl/Determine Control algorithm/DCM to quaternion2 ==
  DCM : Inport
  Abs : Abs  SaturateOnIntegerOverflow=off
  Constant : Constant
  Demux : Demux
  Direction Cosine Matrix to Quaternions1 : sharedtransform/Direction Cosine Matrix  to Quaternions  aMode=0  action=None  tolerance=eps(2)
      settings: LibrarySourceBlock=|
      | aerolibtransform2/Direction Cosine Matrix
      | to Quaternions
  Divide : Product  Inputs=*/
  Extract Diagonal : matrix_library/Extract Diagonal
      settings: LibrarySourceBlock=|
      | simulink/Matrix
      | Operations/Extract Diagonal
  Gain : Gain  Gain=0.5
  Gain1 : Gain  Gain=[0 0 0; 0 0 1; 0 -1 0]
  Gain2 : Gain  Gain=[0 0 -1; 0 0 0; 1 0 0]
  Gain3 : Gain  Gain=[0 1 0; -1 0 0; 0 0 0]
  Gain4 : Gain  Gain=[4;4;4]
  MATLAB Function : MATLAB Function  TreatAsAtomicUnit=on
  Mux : Mux  Inputs=3
  Normalize Vector1 : Subsystem
  Sqrt : Sqrt
  Sum : Sum  Inputs=|++
  Sum of Elements{,1..3} (4 alike) : Sum  Inputs=+
  Unit Delay : UnitDelay  InitialCondition=q0  SampleTime=-1  HasFrameUpgradeWarning=on
  Vector Concatenate : Concatenate  NumInputs=3
  Vector Concatenate1 : Concatenate
  Vector Concatenate2 : Concatenate
  q (scalar last)1 : Outport
  wires:
  Extract Diagonal/1 -> Sum of Elements/1
  Sum of Elements/1 -> Sum/1
  Constant/1 -> Sum/2
  Sqrt/1 -> Gain/1
  DCM/1 -> Gain1/1, Gain2/1, Gain3/1, Extract Diagonal/1
  Gain2/1 -> Sum of Elements1/1
  Sum of Elements1/1 -> Vector Concatenate/2
  Gain1/1 -> Sum of Elements2/1
  Sum of Elements2/1 -> Vector Concatenate/1
  Sum of Elements3/1 -> Vector Concatenate/3
  Gain3/1 -> Sum of Elements3/1
  Vector Concatenate/1 -> Divide/1
  Gain/1 -> Vector Concatenate1/2, Gain4/1
  Divide/1 -> Vector Concatenate1/1
  Vector Concatenate1/1 -> Normalize Vector1/1(Vector)
  Sum/1 -> Abs/1
  Gain4/1 -> Divide/2
  Abs/1 -> Sqrt/1
  Direction Cosine Matrix to Quaternions1/1 -> Demux/1
  Demux/2 -> Mux/1
  Demux/3 -> Mux/2
  Demux/4 -> Mux/3
  Demux/1 -> Vector Concatenate2/2
  Mux/1 -> Vector Concatenate2/1
  Vector Concatenate2/1 -> ?
  ? -> Direction Cosine Matrix to Quaternions1/1
  Unit Delay/1 -> MATLAB Function/2(quat_last)
  MATLAB Function/1(quat) -> Unit Delay/1, q (scalar last)1/1
  Normalize Vector1/1(Versor) -> MATLAB Function/1("quat ")

== system SAD_testControl/Determine Control algorithm/Relative attitude error quaternion3 ==
  q1 (usually Estimated) : Inport
  q2 (Target) : Inport  Port=2
  Demux : Demux
  Gain1 : Gain  Gain=[0,0,0,-1; 0,0,1,0; 0,-1,0 0; 1,0,0,0]
  Gain2 : Gain  Gain=[0, 0, -1 ,0; 0, 0 ,0 ,-1; 1, 0, 0, 0; 0 1, 0, 0]
  Gain3 : Gain  Gain=[0 1 0 0; -1 0 0 0; 0 0 0 -1; 0 0 1 0]
  Gain4 : Gain  Gain=eye(4)
  Matrix Multiply : Product  Multiplication=Matrix(*)
  Sum1 : Sum  Inputs=++++
  qe : Outport
  wires:
  Gain1/1 -> Sum1/1
  Demux/2 -> Gain2/1
  Gain3/1 -> Sum1/3
  Demux/1 -> Gain1/1
  Sum1/1 -> Matrix Multiply/1
  Demux/3 -> Gain3/1
  Gain4/1 -> Sum1/4
  Gain2/1 -> Sum1/2
  Demux/4 -> Gain4/1
  q2 (Target)/1 -> Matrix Multiply/2
  Matrix Multiply/1 -> qe/1
  q1 (usually Estimated)/1 -> Demux/1

== system SAD_testControl/Dynamics e Kinematics/Attitude error GG ==
  w : Inport
  DCM_B/N : Inport  Port=2
  Clock : Clock
  Constant : Constant  Value=n_e
  Constant5 : Constant  Value=0
  Matrix Multiply1 : Product  Multiplication=Matrix(*)
  Product : Product
  Subtract : Sum  Inputs=+-
  Vector Concatenate3 : Concatenate  NumInputs=3
  calculating A_B/L : Subsystem
  Ang Vel Error : Outport
  DCM_B/L : Outport  Port=2
  A_L/N : Outport  Port=3
  wires:
  Constant5/1 -> Vector Concatenate3/2, Vector Concatenate3/1
  Vector Concatenate3/1 -> Matrix Multiply1/2  "w_L/N"
  calculating A_B/L/1(A_B/L) -> Matrix Multiply1/1, DCM_B/L/1
  Matrix Multiply1/1 -> Subtract/2  "A_B/L * w_L/N"
  w/1 -> Subtract/1
  Subtract/1 -> Ang Vel Error/1
  Product/1 -> calculating A_B/L/1(Theta)  "Theta"
  Clock/1 -> Product/2
  Constant/1 -> Product/1, Vector Concatenate3/3
  DCM_B/N/1 -> calculating A_B/L/2(A_B/N)
  calculating A_B/L/2(A_L/N) -> A_L/N/1

== system SAD_testControl/Dynamics e Kinematics/DCM composition from quaternions 1 ==
  q(4x1) : Inport
  Cross product matrix composition : Subsystem
  Demux : Demux
  Dot Product : DotProduct  OutDataTypeStr=Inherit: Inherit via internal rule
  Gain : Gain  Gain=[1 0 0; 0 1 0; 0 0 1]
  Gain1 : Gain  Gain=2
  Gain2 : Gain  Gain=-2
  Mux : Mux  Inputs=3
  Product : Product  Multiplication=Matrix(*)
  Product1 : Product
  Square : Math  Operator=square
  Sum : Sum  Inputs=|-+
  Sum1 : Sum  Inputs=+++
  Transpose : Math  Operator=transpose
  DCM : Outport
  wires:
  Gain/1 -> Sum1/1
  Demux/1 -> Mux/1
  q(4x1)/1 -> Demux/1
  Demux/2 -> Mux/2
  Mux/1 -> Dot Product/2, Dot Product/1, Product/1, Cross product matrix composition/1(q_vect), Transpose/1  "q_vect"
  Demux/4 -> Gain2/1, Square/1  "q4"
  Demux/3 -> Mux/3
  Dot Product/1 -> Sum/1
  Sum/1 -> Gain/1
  Square/1 -> Sum/2
  Transpose/1 -> Product/2
  Product/1 -> Gain1/1
  Gain2/1 -> Product1/2
  Cross product matrix composition/1(q_vect cross) -> Product1/1  "omega_mat"
  Product1/1 -> Sum1/3
  Gain1/1 -> Sum1/2
  Sum1/1 -> DCM/1

== system SAD_testControl/Dynamics e Kinematics/Kinematics quaternion2 ==
  omega : Inport
  q0 : Inport  Port=2
  Demux : Demux
  Divide : Product  Inputs=*/
  Gain1 : Gain  Gain=-1
  Gain2 : Gain  Gain=-1
  Gain3 : Gain  Gain=1/2
  Gain4 : Gain  Gain=-1
  Integrator : Integrator  InitialConditionSource=external
  Matrix Multiply : Product  Multiplication=Matrix(*)
  Matrix OMEGA : Subsystem
  Mux : Mux
  Normalize Vector2 : Subsystem
  q : Outport
  q^(-1) : Outport  Port=2
  wires:
  Gain3/1 -> Matrix Multiply/1
  Matrix Multiply/1 -> Integrator/1
  omega/1 -> Matrix OMEGA/1(omega)
  Integrator/1 -> Normalize Vector2/1(Vector), Divide/1, Demux/1, q/1
  Matrix OMEGA/1(Matrix Omega) -> Gain3/1
  q0/1 -> Integrator/2
  Demux/2 -> Gain1/1
  Demux/3 -> Gain2/1
  Demux/4 -> Gain4/1
  Gain1/1 -> Mux/2
  Gain2/1 -> Mux/3
  Gain4/1 -> Mux/4
  Demux/1 -> Mux/1
  Mux/1 -> q^(-1)/1
  Normalize Vector2/1(Norm) -> Divide/2
  Divide/1 -> Matrix Multiply/2
